simulink model "simulink_model_test_bms"  (R2016a)
settings: Solver=ode23tb  StartTime=357510  StopTime=372620  MaxStep=1  RelTol=1e-4
undefined symbols (not defined in the file or in its folder): Ion, Lithium
libraries: powerlib x6, electricdrivelib x1
Description:
  | Copyright 2008-2016 The MathWorks, Inc.
settings Model: NumberOfSteps=100  Creator=MathWorks  LastModifiedBy=fkazhami
settings DataIOCC: LimitDataPoints=on  SaveFormat=Array
settings OptimizationCC: ExpressionDepthLimit=2147483647  InitFltsAndDblsToZero=on
settings DebuggingCC: UnderspecifiedInitializationDetection=Classic  MergeDetectMultiDrivingBlocksExec=none  SignalResolutionControl=TryResolveAllWithWarning  SolverPrmCheckMsg=warning  FcnCallInpInsideContextMsg=UseLocalSettings  AllowSymbolicDim=off  StateNameClashWarn=warning
settings HardwareCC: ProdBitPerPointer=32  ProdLargestAtomicFloat=None  ProdIntDivRoundTo=Undefined  ProdEndianess=Unspecified  ProdWordSize=32  ProdHWDeviceType=32-bit Generic
settings ModelReferenceCC: PropagateSignalLabelsOutOfModel=off
settings GRTTargetCC: CombineOutputUpdateFcns=off  GRTInterface=on
settings ConfigComp: CovModelRefEnable=Off

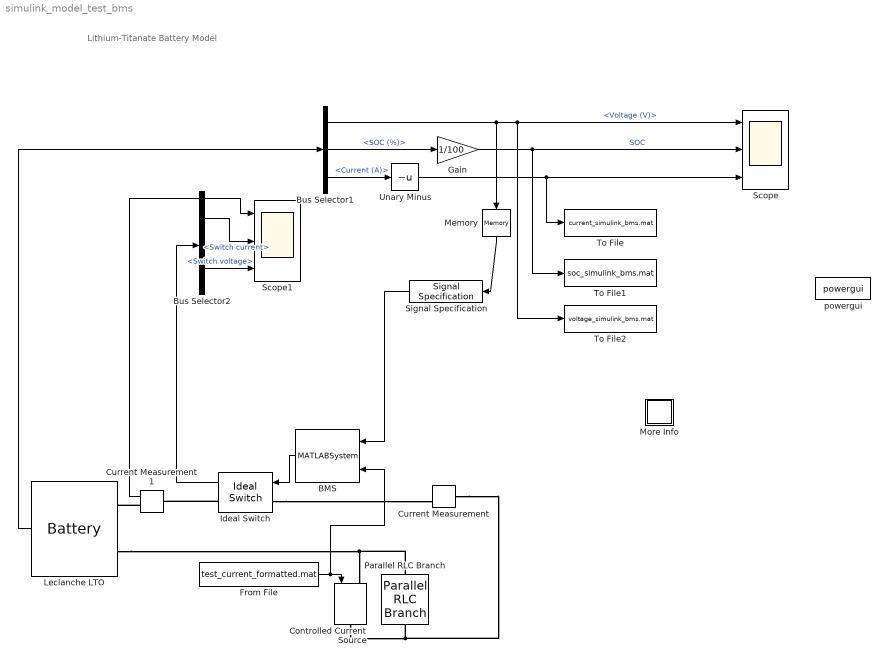
== system simulink_model_test_bms ==
  note: Lithium-Titanate Battery Model
  BMS : MATLABSystem  System=simple_bms  Vmin=1.5  Vmax=2.7  SimulateUsing=Code generation
      mask Type: simple_bms
      mask Display:
      | disp('simple_bms');
      | port_label('input',1,'voltage');
      | port_label('input',2,'current');
      | port_label('output',1,'y');
  Bus Selector1 : BusSelector  OutputSignals=Voltage (V),SOC (%),Current (A)
  Bus Selector2 : BusSelector  OutputSignals=Switch current,Switch voltage
  Controlled Current Source : powerlib/Electrical Sources/Controlled Current Source  Initialize=on  Source_Type=DC  Amplitude=0  Phase=0  Frequency=0  Measurements=None
  Current Measurement : powerlib/Measurements/Current Measurement  PhasorSimulation=off  OutputType=Complex  PSBequivalent=0
  Current Measurement1 : powerlib/Measurements/Current Measurement  PhasorSimulation=off  OutputType=Complex  PSBequivalent=0
  From File : FromFile  FileName=test_current_formatted.mat  SampleTime=10
  Gain : Gain  Gain=1/100
  Ideal Switch : powerlib/Power Electronics/Ideal Switch  Ron=0.001  Lon=0  IC=1  Rs=inf  Cs=0  Measurements=on
  Leclanche LTO : electricdrivelib/Extra Sources/Battery  BatType=Lithium-Ion  ShowTempParam=off  ThermalPreset=no  NomV=1.95  NomQ=30  SOC=9  Batt_Tr=30  PresetModel=off  MaxQ=32  MinV=1.5  FullV=2.7  Dis_rate=30  R=0.002  Normal_OP=25  expZone="[2.5      1]"  current=[50 100 150]  Units=Ampere-hour  Tci=20  NomT=25  T2=0  MaxQ2=2.208  FullV2=3.45  Normal_OP2=2.8  expZone2="[3.22        0.23]"  Rca=0.6  ti=1000  Dp=0
  Memory : Memory  X0=1.95  LinearizeAsDelay=on
  More Info : Subsystem
      settings: OpenFcn=showdemo(bdroot(gcb))
      mask Display: disp('?')
  Parallel RLC Branch : powerlib/Elements/Parallel RLC Branch  LConnTagsString=a  RConnTagsString=__new0  BranchType=R  Resistance=1e6  Inductance=0  SetiL0=off  InitialCurrent=0  Capacitance=1e-6  Setx0=off  InitialVoltage=0  Measurements=None
  Scope : Scope  NumInputPorts=3
  Scope1 : Scope  NumInputPorts=3
  Signal Specification : SignalSpecification  OutMin=[0]  OutMax=[1000]  Dimensions=[1]
  To File : ToFile  Filename=current_simulink_bms.mat  MatrixName=c  SampleTime=10
  To File1 : ToFile  Filename=soc_simulink_bms.mat  MatrixName=soc  SampleTime=10
  To File2 : ToFile  Filename=voltage_simulink_bms.mat  MatrixName=v  SampleTime=2
  Unary Minus : UnaryMinus
  powergui : powerlib/powergui  SimulationMode=Discrete  SolverType=Tustin  SampleTime=2  frequency=60  SPID=off  DisableSnubberDevices=off  DisableRonSwitches=off  DisableVfSwitches=off  SwTol=0  DisplayEquations=off  Interpol=off  ExternalGateDelay=off  methode=off  Ts=0  FunctionMessages=off  echomessages=off  HookPort=off  EnableUseOfTLC=off  x0status=blocks  frequencyindice=0  Pbase=100e6  ErrMax=1e-4  Iterations=50  UnitsV=V  UnitsW=W  buscounter=0  RestoreLinks=warning  ResistiveCurrentMeasurement=off  Frange=[0:2:500]  Ylog=off  Xlog=on  ShowGrid=off  save=off  variable=ZData  structure=0  ZoomFFT=on  StartTime=0.0  cycles=1  DisplayStyle=1  fundamental=60  FreqAxis=off  MaxFrequency=1000  frequencyindicesteady=1  RmsSteady=1  display=off
  wires:
  Leclanche LTO/1 -> Bus Selector1/1
  Bus Selector1/2 -> Gain/1  "<SOC (%)>"
  Gain/1 -> To File1/1, Scope/2  "SOC"
  Bus Selector1/3 -> Unary Minus/1  "<Current (A)>"
  From File/1 -> BMS/2, Controlled Current Source/1
  Unary Minus/1 -> To File/1, Scope/3
  Bus Selector1/1 -> To File2/1, Scope/1, Memory/1  "<Voltage (V)>"
  BMS/1 -> Ideal Switch/1
  Memory/1 -> Signal Specification/1
  Signal Specification/1 -> BMS/1
  Ideal Switch/1 -> Bus Selector2/1
  Bus Selector2/2 -> Scope1/3  "<Switch voltage>"
  Bus Selector2/1 -> Scope1/2  "<Switch current>"
  Current Measurement1/1 -> Scope1/1
  connections:
  Leclanche LTO/LConn2 -- Controlled Current Source/LConn1 -- Parallel RLC Branch/LConn1
  Controlled Current Source/RConn1 -- Current Measurement/LConn1 -- Parallel RLC Branch/RConn1
  Ideal Switch/LConn1 -- Current Measurement/RConn1
  Current Measurement1/RConn1 -- Leclanche LTO/LConn1
  Ideal Switch/RConn1 -- Current Measurement1/LConn1

== system simulink_model_test_bms/More Info ==
